simulink model "modelPredictiveControl_v0"  (R2024b)
settings: Solver=FixedStepAuto  StartTime=0.0  StopTime=80  FixedStep=0.01  RelTol=1e-3
undefined symbols (not defined in the file or in its folder): C, del_t, initial_conditions
libraries: mpclib x3
(part 2 of 2)

== matlab function modelPredictiveControl_v0/Pendulum-Cart (Tracking)/MATLAB Function2 ==
  data: r input; A input; delta_U output; B input; C input; x_k input; y_k input; previous_u input; previous_x input
function delta_U = MPC(r, A, B, C, x_k, y_k, previous_u, previous_x)
    coder.extrinsic("quadprog");
    lx = 4;
    ly = 2;
    lu = 1;
    Nx = 40;    % Prediction horizon
    Nu = 10;     % Control horizon

    %% --------------------------------------------------------------------
    % Construct Ge = 2(upsilon + (gamma)' xi gamma)    
    % upsilon
    R = 0.005*eye(lu);   % Cost weight for change in input (delta u)
    upsilon = kron(eye(Nu), R);

    % xi
    Q = [5 0;0 20];    % Cost weight for state
    P = Q;%1*eye(ly);
    xi = kron(eye(Nx-1), Q);
    xi = blkdiag(xi, P);

    % gamma
    Ce = [zeros(ly,lx) eye(ly)];
    Be = zeros(lx+ly, lu);
    % Be(1:lx, 1:lu) = B;
    % Be((lx+1):(lx+ly), 1:lu) = C*B;
    Be = [B; C*B];
    Ae = zeros(lx+ly);
    Ae(1:lx, 1:lx) = A;
    Ae((lx + 1):(lx + ly), 1:lx) = C*A;
    Ae((lx + 1):(lx + ly), (lx + 1):(lx + ly)) = eye(ly);

    gamma_first_col = zeros(Nx*ly, lu);
    % Create the first column of gamma, i.e., [CeBe CeAeBe ... CeAe^(Nx-1)Be]'
    for i = 0:(Nx-1)
        j = Ce * Ae^i * Be;
        gamma_first_col((i*ly + 1):((i+1)*ly), 1:lu) = j;
    end
    % Fill up rest of the gamma
    gamma = [gamma_first_col zeros(Nx*ly, (Nu-1)*lu)];
    for i = 1:(Nu-1)
        j = gamma_first_col(1:(Nx-i)*ly, 1:lu);
        gamma((i*ly + 1):(Nx*ly), (i*lu + 1):((i+1)*lu)) = j;
    end

    % Ge
    Ge = 2 * (upsilon + transpose(gamma) * xi * gamma);
    %% --------------------------------------------------------------------

    %% --------------------------------------------------------------------
    % Construct X = [delta_x  y]', Te = [X  previous_u  r]'

    % X
    delta_x = x_k - previous_x;
    X = [delta_x;
         y_k];

    % Te
    Te = zeros(lx + ly + lu + Nx*ly, 1);
    Te(1:(lx + ly)) = X;
    Te((lx + ly + 1):(lx + ly + lu)) = previous_u;
    Te((lx + ly + lu + 1):end) = r;
    % Te = [X;
    %       previous_u;
    %       r];
    %% --------------------------------------------------------------------

    %% --------------------------------------------------------------------
    % Construct eF = [2 (phi)' xi gamma    0    -2 xi gamma]'
    % where phi = [CeAe ... CeAe^(Nx)]'

    % phi
    phi = zeros(Nx*ly, (lx + ly));
    for i = 1:Nx
        phi(((i-1)*ly + 1):i*ly, 1:(lx + ly)) = Ce*Ae^i;
    end

    % eF
    eF = [2 * transpose(phi) * xi * gamma;
          zeros(lu, Nu*lu);
         -2 * xi * gamma];
    %% --------------------------------------------------------------------

    %% --------------------------------------------------------------------
    % Construct J = [-L  L  -I  I  gamma  -gamma]'

    % L
    lower_triangluar_ones = tril(ones(Nu));
    L = kron(lower_triangluar_ones, eye(lu));

    % J
    J = [-L;
          L;
         -eye(Nu*lu);
          eye(Nu*lu);
          gamma;
         -gamma];
    %% --------------------------------------------------------------------

    %% --------------------------------------------------------------------
    % Construct Wo = [-u0_min ... -u(Nu-1)_min  u0_max ... u(Nu-1)_max
    %                 -delta_u0_min ... -delta_u(Nu-1)_min  delta_u0_max ... delta_u(Nu-1)_max
    %                 -e1_min ... -e(Nx)_min  e1_max ... e(Nx)_max]'

    % Constraints on u
    u_min = [-75];
    u_max = [75];
    Wo_upper_block = [kron(-ones(Nu,1), u_min); kron(ones(Nu,1), u_max)];

    % Constraints on delta u
    delta_u_min = [-50];
    delta_u_max = [50];
    Wo_middle_block = [kron(-ones(Nu,1), delta_u_min); kron(ones(Nu,1), delta_u_max)];

    % Constraints on tracking error
    e_min = [-10;
             -200];
    e_max = [10;
             200];
    Wo_lower_block = [kron(-ones(Nx,1), e_min); kron(ones(Nx,1), e_max)];

    Wo = [Wo_upper_block; Wo_middle_block; Wo_lower_block];
    %% --------------------------------------------------------------------

    %% --------------------------------------------------------------------
    % Construct eX
    
    % iota
    iota = kron(ones(Nu,1), eye(lu));

    % eX
    % eX = zeros(4*Nu*lu + 2*Nx*ly, lx + ly + lu + Nx*ly);
    % eX((4*Nu*lu + 1):(4*Nu*lu + Nx*ly), 1:(lx + ly)) = -phi;
    % eX((4*Nu*lu + 1 + Nx*ly):(4*Nu*lu + 2*Nx*ly), 1:(lx + ly)) =  phi;
    % 
    % eX(1:(Nu*lu), (lx + ly + 1):(lx + ly + lu)) = iota;
    % eX((Nu*lu + 1):(2*Nu*lu), (lx + ly + 1):(lx + ly + lu)) = -iota;
    % 
    % eX((4*Nu*lu + 1):(4*Nu*lu + Nx*ly), (lx + ly + lu + 1):(lx + ly + lu + Nx*ly)) = -eye(Nx*ly);
    % eX((4*Nu*lu + 1 + Nx*ly):(4*Nu*lu + 2*Nx*ly), (lx + ly + lu + 1):(lx + ly + lu + Nx*ly)) = eye(Nx*ly);

    eX = [zeros(Nu*lu, lx+ly), iota, zeros(Nu*lu, Nx*ly);
          zeros(Nu*lu, lx+ly), -iota, zeros(Nu*lu, Nx*ly);
          zeros(2*Nu*lu, lx+ly + lu + Nx*ly);
          -phi, zeros(Nx*ly, lu), -eye(Nx*ly);
          phi, zeros(Nx*ly, lu), eye(Nx*ly)];
    %% --------------------------------------------------------------------

    %% --------------------------------------------------------------------
    % Setting up quadprog
    b = Wo + eX * Te;
    f = transpose(Te) * eF;
    delta_U = zeros(Nu*lu, 1);
    delta_U = quadprog(Ge,f,J,b);
    %% --------------------------------------------------------------------

end

== matlab function modelPredictiveControl_v0/Pendulum-Cart (Tracking)/MATLAB Function4 ==
  data: delta_U input; u output; previous_u input
function u = first_u(delta_U, previous_u)
    lu = 1;
    u = previous_u + delta_U(1:lu);
end

== matlab function modelPredictiveControl_v0/Pendulum-Cart (Tracking Unconstrained)/MATLAB Function ==
  data: x input; u input; A output; B output; C output; x_k output; y_k output
function [A, B, C, x_k, y_k] = discrete_pendulum_cart_model(x, u)
    coder.extrinsic('ss');
    coder.extrinsic("c2d");
    coder.extrinsic("ssdata");
    % Physical Parameters
    m1 = 1; m2 = 1; ell = 0.1; k = 0; g = 9.81; kappa = 0;

    % Continuous-time model
    Ac = [0 1 0 0;
          k/(m1 + m2 - m2 * cos(x(3))^2) 0 (2*m2*cos(x(3))*ell^2*x(4)^2 + 2*g*m2*cos(2*x(3))*ell + 2*kappa*cos(x(3)) - 2*kappa*x(3)*sin(x(3)))/(ell*(2*m1 + m2 - m2*cos(2*x(3)))) - (4*u*m2*sin(2*x(3)))/(2*m1 + m2 - m2*cos(2*x(3)))^2 - (4*m2*sin(2*x(3))*(kappa*x(3)*cos(x(3)) + ell*k*x(1) + ell^2*m2*x(4)^2*sin(x(3)) + (ell*g*m2*sin(2*x(3)))/2))/(ell*(2*m1 + m2 - m2*cos(2*x(3)))^2) (2*ell*m2*x(4)*sin(x(3)))/(m2*sin(x(3))^2 + m1);
          0 0 0 1;
          -(k*cos(x(3)))/(ell*(- m2*cos(x(3))^2 + m1 + m2)) 0 (ell^2*m2^3*x(4)^2 - kappa*m2^2 - 2*kappa*m1*m2 - kappa*m1^2 + kappa*m2^2*cos(x(3))^2 - ell*g*m2^3*cos(x(3))^3 + ell^2*m1*m2^2*x(4)^2 - ell*u*m2^2*sin(x(3))^3 + kappa*m2^2*x(3)*sin(2*x(3)) + ell*g*m2^3*cos(x(3)) + kappa*m1*m2*cos(x(3))^2 + 2*ell*u*m2^2*sin(x(3)) - ell^2*m2^3*x(4)^2*cos(x(3))^2 - ell*g*m1^2*m2*cos(x(3)) + 2*ell*k*m2^2*x(1)*sin(x(3)) + kappa*m1*m2*x(3)*sin(2*x(3)) - 2*ell^2*m1*m2^2*x(4)^2*cos(x(3))^2 - ell*g*m1*m2^2*cos(x(3))^3 - ell*k*m2^2*x(1)*sin(x(3))^3 + ell*u*m1*m2*sin(x(3)) + ell*k*m1*m2*x(1)*sin(x(3)))/(ell^2*m2*(- m2*cos(x(3))^2 + m1 + m2)^2) -(2*m2*x(4)*sin(2*x(3)))/(2*m1 + m2 - m2*cos(2*x(3)))];
    Bc = [0;
          1/(m1 + m2 - m2 * cos(x(3))^2);
          0;
          (-cos(x(3))/ell) * (1/(m1 + m2 - m2 * cos(x(3))^2))];
    Cc = [1 0 0 0;
          0 0 1 0];
    % Cc = [0 0 1 0];
    Dc = [0; 0];

    % % Discrete-time model Method 1
    % del_t = 0.01;
    % nx = size(Ac, 1);
    % nu = size(Bc, 2);
    % M = expm([[Ac Bc]*del_t; zeros(nu, nx+nu)]);
    % A = M(1:nx, 1:nx);
    % B = M(1:nx, nx+1:nx+nu);
    % C = Cc;
    % D = Dc;

    % Discrete-time model Method 2
    % Preinitializing the sizes of Ad, Bd, Cd, Dd
    A = Ac; B = Bc; C = Cc; D = Dc;
    % Discretization
    del_t = 0.01;
    [A, B, C, D] = ssdata(c2d(ss(Ac,Bc,Cc,Dc),del_t));
    x_k = x;
    y_k = C*x_k;
end

== matlab function modelPredictiveControl_v0/Pendulum-Cart (Tracking Unconstrained)/r(k) ==
  data: t input; r output
function r = reference_trajectory(t)
    N_x = 40;
    set_point = [3; deg2rad(180)];
    if (t > 25)
        set_point = [-3; deg2rad(180)];
    end
    r = kron(ones(N_x, 1), set_point);
end

== matlab function modelPredictiveControl_v0/Pendulum-Cart (Tracking)/r(k) ==
  data: t input; r output
function r = reference_trajectory(t)
    N_x = 40;
    set_point = [3; deg2rad(180)];
    %if (t > 25)
    %    set_point = [-3; deg2rad(180)];
    %end

    if (t < 10)
        set_point = [3; deg2rad(180)];
    elseif (t < 30)
        set_point = [0; deg2rad(180)];
    elseif (t < 60)
        set_point = [-2; deg2rad(180)];
    else
        set_point = [0; deg2rad(180)];
    end

    r = kron(ones(N_x, 1), set_point);
end

== matlab function modelPredictiveControl_v0/Pendulum-Cart (Tracking)/MATLAB Function5 ==
  data: x input; u input; x_dot output
function x_dot = pendulum_cart_dynamics(x, u)
    m1 = 1; m2 = 1; l = 0.1; k = 0; g = 9.81; kappa = 0;

    f_x_1 = x(2);
    f_x_2 = 1/(m1 + m2 - m2 * (cos(x(3)))^2) * ...
             (m2 * g * sin(x(3)) * cos(x(3)) + (kappa/l) * cos(x(3)) * x(3) + ...
             k * x(1) + m2 * l * sin(x(3)) * x(4)^2);
    f_x_3 = x(4);
    f_x_4 = f_x_2 * (-cos(x(3))/l) - (g/l) * sin(x(3)) - ...
             (kappa/(m2*l^2)) * x(3);
    f_x = [f_x_1; f_x_2; f_x_3; f_x_4];
    
    g_x = [0;
           1/(m1 + m2 - m2 * cos(x(3))^2);
           0;
           (-cos(x(3))/l) * (1/(m1 + m2 - m2 * cos(x(3))^2))];

    x_dot = f_x + g_x * u;
end

== matlab function modelPredictiveControl_v0/Simple Pendulum (Tracking)/Plant ==
  data: x input; u input; x_dot output
function x_dot = pendulum_dynamics(x, u)
    g = 9.81; l = 1;
    x_dot = [x(2);
             -(g/l) * sin(x(1)) + (1/l) * u];
end

== matlab function modelPredictiveControl_v0/Pendulum-Cart (Tracking)/MATLAB Function7 ==
  data: x input; x output
function x = rad_to_deg(x)
    x(3) = rad2deg(x(3));
    x(4) = rad2deg(x(4));
end

== matlab function modelPredictiveControl_v0/Mass System (Stabilization)/Plant ==
  data: x input; u input; x_dot output
function x_dot = simple_mass_system(x, u)
    A = [0 1; 0 0];
    B = [0; 1];

    x_dot = A*x + B*u;
end

== matlab function modelPredictiveControl_v0/Simple Pendulum (Toolbox)(Doesn't Work)/MATLAB Function1 ==
  data: t input; x_d output
function x_d = desired_trajectory(t)
    x_d = -deg2rad(180);
    if t < 2
        x_d = deg2rad(180);
    end
    x_d = deg2rad(180);
end

== matlab function modelPredictiveControl_v0/Simple Pendulum (Toolbox)(Doesn't Work)/MATLAB Function ==
  data: x input; u input; x_dot output
function x_dot = pendulum_dynamics(x, u)
    g = 9.81; l = 1;
    x_dot = [x(2);
             -(g/l) * sin(x(1)) + (1/l) * u];
end

== matlab function modelPredictiveControl_v0/Pendulum-Cart (Tracking Unconstrained)/MATLAB Function2 ==
  data: r input; A input; delta_U output; B input; C input; x_k input; y_k input; previous_u input; previous_x input
function delta_U = MPC(r, A, B, C, x_k, y_k, previous_u, previous_x)
    coder.extrinsic("quadprog");
    lx = 4;
    ly = 2;
    lu = 1;
    Nx = 40;    % Prediction horizon
    Nu = 10;     % Control horizon

    %% --------------------------------------------------------------------
    % Construct Ge = 2(upsilon + (gamma)' xi gamma)    
    % upsilon
    R = 0.005*eye(lu);   % Cost weight for change in input (delta u)
    upsilon = kron(eye(Nu), R);

    % xi
    Q = [5 0;0 20];    % Cost weight for state
    P = Q;%1*eye(ly);
    xi = kron(eye(Nx-1), Q);
    xi = blkdiag(xi, P);

    % gamma
    Ce = [zeros(ly,lx) eye(ly)];
    Be = zeros(lx+ly, lu);
    % Be(1:lx, 1:lu) = B;
    % Be((lx+1):(lx+ly), 1:lu) = C*B;
    Be = [B; C*B];
    Ae = zeros(lx+ly);
    Ae(1:lx, 1:lx) = A;
    Ae((lx + 1):(lx + ly), 1:lx) = C*A;
    Ae((lx + 1):(lx + ly), (lx + 1):(lx + ly)) = eye(ly);

    gamma_first_col = zeros(Nx*ly, lu);
    % Create the first column of gamma, i.e., [CeBe CeAeBe ... CeAe^(Nx-1)Be]'
    for i = 0:(Nx-1)
        j = Ce * Ae^i * Be;
        gamma_first_col((i*ly + 1):((i+1)*ly), 1:lu) = j;
    end
    % Fill up rest of the gamma
    gamma = [gamma_first_col zeros(Nx*ly, (Nu-1)*lu)];
    for i = 1:(Nu-1)
        j = gamma_first_col(1:(Nx-i)*ly, 1:lu);
        gamma((i*ly + 1):(Nx*ly), (i*lu + 1):((i+1)*lu)) = j;
    end

    % Ge
    Ge = 2 * (upsilon + transpose(gamma) * xi * gamma);
    %% --------------------------------------------------------------------

    %% --------------------------------------------------------------------
    % Construct X = [delta_x  y]'

    % X
    delta_x = x_k - previous_x;
    X = zeros((lx + ly), 1);
    X(1:lx) = delta_x;
    X(lx+1:lx+ly) = y_k;
    %% --------------------------------------------------------------------

    %% --------------------------------------------------------------------
    % Construct RHS = ( -2 (X)' (phi)' xi gamma + 2 r' xi gamma )'

    % phi
    phi = zeros(Nx*ly, (lx + ly));
    for i = 1:Nx
        phi(((i-1)*ly + 1):i*ly, 1:(lx + ly)) = Ce*Ae^i;
    end

    % RHS
    RHS = -2 * transpose(X) * transpose(phi) * xi * gamma + 2 * transpose(r) * xi * gamma;
    RHS = transpose(RHS);
    %% --------------------------------------------------------------------

    %% --------------------------------------------------------------------
    % Setting up quadprog
    delta_U = Ge \ RHS;
    %% --------------------------------------------------------------------

end

== matlab function modelPredictiveControl_v0/Pendulum-Cart (Stabilization)/MATLAB Function ==
  data: x input; u input; A output; B output; x_k output
function [A, B, x_k] = discrete_pendulum_cart_model(x, u)
    coder.extrinsic('ss');
    coder.extrinsic("c2d");
    coder.extrinsic("ssdata");
    % Physical Parameters
    m1 = 1; m2 = 1; ell = 0.1; k = 0; g = 9.81; kappa = 0;

    % Continuous-time model
    Ac = [0 1 0 0;
          k/(m1 + m2 - m2 * cos(x(3))^2) 0 (2*m2*cos(x(3))*ell^2*x(4)^2 + 2*g*m2*cos(2*x(3))*ell + 2*kappa*cos(x(3)) - 2*kappa*x(3)*sin(x(3)))/(ell*(2*m1 + m2 - m2*cos(2*x(3)))) - (4*u*m2*sin(2*x(3)))/(2*m1 + m2 - m2*cos(2*x(3)))^2 - (4*m2*sin(2*x(3))*(kappa*x(3)*cos(x(3)) + ell*k*x(1) + ell^2*m2*x(4)^2*sin(x(3)) + (ell*g*m2*sin(2*x(3)))/2))/(ell*(2*m1 + m2 - m2*cos(2*x(3)))^2) (2*ell*m2*x(4)*sin(x(3)))/(m2*sin(x(3))^2 + m1);
          0 0 0 1;
          -(k*cos(x(3)))/(ell*(- m2*cos(x(3))^2 + m1 + m2)) 0 (ell^2*m2^3*x(4)^2 - kappa*m2^2 - 2*kappa*m1*m2 - kappa*m1^2 + kappa*m2^2*cos(x(3))^2 - ell*g*m2^3*cos(x(3))^3 + ell^2*m1*m2^2*x(4)^2 - ell*u*m2^2*sin(x(3))^3 + kappa*m2^2*x(3)*sin(2*x(3)) + ell*g*m2^3*cos(x(3)) + kappa*m1*m2*cos(x(3))^2 + 2*ell*u*m2^2*sin(x(3)) - ell^2*m2^3*x(4)^2*cos(x(3))^2 - ell*g*m1^2*m2*cos(x(3)) + 2*ell*k*m2^2*x(1)*sin(x(3)) + kappa*m1*m2*x(3)*sin(2*x(3)) - 2*ell^2*m1*m2^2*x(4)^2*cos(x(3))^2 - ell*g*m1*m2^2*cos(x(3))^3 - ell*k*m2^2*x(1)*sin(x(3))^3 + ell*u*m1*m2*sin(x(3)) + ell*k*m1*m2*x(1)*sin(x(3)))/(ell^2*m2*(- m2*cos(x(3))^2 + m1 + m2)^2) -(2*m2*x(4)*sin(2*x(3)))/(2*m1 + m2 - m2*cos(2*x(3)))];
    Bc = [0;
          1/(m1 + m2 - m2 * cos(x(3))^2);
          0;
          (-cos(x(3))/ell) * (1/(m1 + m2 - m2 * cos(x(3))^2))];
    Cc = [1 0 0 0;
          0 0 1 0];
    Dc = [0; 0];

    % % Discrete-time model Method 1
    % del_t = 0.01;
    % nx = size(Ac, 1);
    % nu = size(Bc, 2);
    % M = expm([[Ac Bc]*del_t; zeros(nu, nx+nu)]);
    % A = M(1:nx, 1:nx);
    % B = M(1:nx, nx+1:nx+nu);
    % C = Cc;
    % D = Dc;

    % Discrete-time model Method 2
    % Preinitializing the sizes of Ad, Bd, Cd, Dd
    A = Ac; B = Bc; C = Cc; D = Dc;
    % Discretization
    del_t = 0.01;
    [A, B, C, D] = ssdata(c2d(ss(Ac,Bc,Cc,Dc),del_t));
    x_k = x;
end

== matlab function modelPredictiveControl_v0/Simple Pendulum (Toolbox)(Doesn't Work)/MATLAB Function2 ==
  data: del_t input; x input; u input; A output; B output; C output; D output; U output; Y output; X output; DX output
function [A, B, C, D, U, Y, X, DX] = discrete_pendulum_model(del_t, x, u)
    % Linearize at each operating point and discretize the linear model

    % Physical Parameters
    g = 9.81; ell = 1;

    % Linearized Model
    Ac = [0 1;
         -(g/ell) * cos(x(1)) 0];
    Bc = [0; 1/ell];
    Cc = [1 0];
    Dc = [0];

    % Discretized Model
    nx = size(Ac, 1);
    nu = size(Bc, 2);
    M = expm([[Ac Bc]*del_t; zeros(nu, nx+nu)]);
    A = M(1:nx, 1:nx);
    B = M(1:nx, nx+1:nx+nu);
    C = Cc;
    D = Dc;

    % [A, B, C, D] = ssdata(c2d(ss(Ac,Bc,Cc,Dc),del_t));

    % Plant nominal conditions
    X = x;
    U = u;
    Y = C*X + D*U;
    DX = A*X + B*U - X;
end
